simulink model "Analog_Digital_PID"  (R2025b)
settings: Solver=FixedStepAuto  StartTime=0.0  StopTime=inf  RelTol=1e-3  EnableMultiTasking=on
libraries: arduinolib x1, arduinoavrlib x1
settings Model: ExtModeTrigDuration=2  Creator=MSI  LastModifiedBy=MSI
settings SolverCC: AutoInsertRateTranBlk=on
settings OptimizationCC: EnhancedBackFolding=on  PassReuseOutputArgsAs=Individual arguments  ZeroExternalMemoryAtStartup=off  ZeroInternalMemoryAtStartup=off  MaxStackSize=64  OptimizeBlockOrder=speed  DifferentSizesBufferReuse=on  OptimizationCustomize=off  EfficientTunableParamExpr=on
settings DebuggingCC: ParameterTunabilityLossMsg=error
settings HardwareCC: ProdBitPerInt=16.0  ProdBitPerPointer=16.0  ProdBitPerSizeT=16.0  ProdBitPerPtrDiffT=16.0  ProdLargestAtomicFloat=None  ProdWordSize=8.0  ProdHWDeviceType=Atmel->AVR
settings SFSimCC: MATLABDynamicMemAlloc=off
settings RTWCC: SystemTargetFile=ert.tlc  HardwareBoard=Arduino Uno  TemplateMakefile=ert_default_tmf  Toolchain=Arduino AVR  BuildConfiguration=Faster Runs  Description=Embedded Coder
settings CodeAppCC: ForceParamTrailComments=on  IgnoreCustomStorageClasses=off  OperatorAnnotations=on  SimulinkDataObjDesc=on  SFDataObjDesc=on  InsertBlockDesc=on
settings ERTTargetCC: ExtModeTransport=3.0  ExtModeStaticAlloc=on  ExtModeAutomaticAllocSize=off  ExtModeStaticAllocSize=250.0  ExtModeMexFile=ext_xcp  ExtModeIntrfLevel=Level2 - Open  InlinedParameterPlacement=Hierarchical  SupportContinuousTime=on  SupportVariableSizeSignals=on

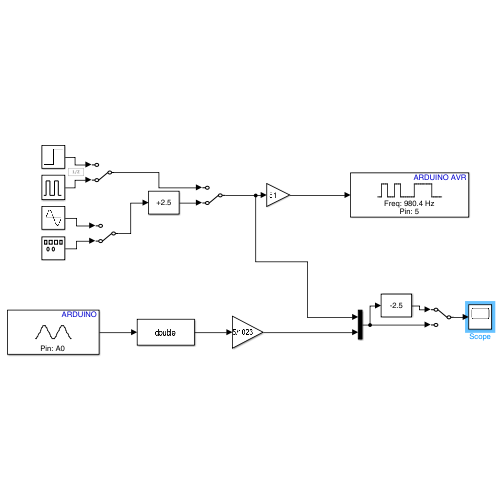
[thumbnail: Simulink's stored preview of the top-level diagram]
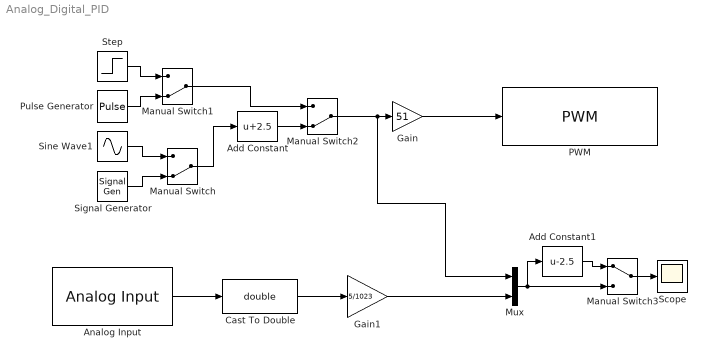
== system Analog_Digital_PID ==
  Add Constant : Bias  Bias=2.5  SaturateOnIntegerOverflow=off
  Add Constant1 : Bias  Bias=-2.5  SaturateOnIntegerOverflow=off
  Analog Input : arduinolib/Analog Input  pinNumber=0  ReadResultsOnly=off  ConversionTriggerSource=Software  ExternalTriggerType=uint32( 0 )  OutputDataType=uint16  EnableConversionCompleteNotify=off  EnableOuputStatus=off  SampleTime=0.01  blockPlatform=arduino
  Cast To Double : DataTypeConversion  OutDataTypeStr=double  SaturateOnIntegerOverflow=off  RndMeth=Floor
  Gain : Gain  Gain=51
  Gain1 : Gain  Gain=5/1023
  Manual Switch : ManualSwitch  CurrentSetting=0
  Manual Switch1 : ManualSwitch  CurrentSetting=0
  Manual Switch2 : ManualSwitch  CurrentSetting=0
  Manual Switch3 : ManualSwitch
  Mux : Mux  Inputs=2
  PWM : arduinoavrlib/PWM  pinNumber=5  desiredFrequency=980.4  achievableFrequency=980.4  EnableCompareMatchInterrupt=off  EnableOverflowInterrupt=off
  Pulse Generator : DiscretePulseGenerator  PulseType=Time based  Amplitude=5  Period=4  PulseWidth=50
  Scope : Scope
      settings: ActiveDisplayYMinimum=0.54594465242270174  ActiveDisplayYMaximum=1.5449366782755996  DataLoggingVariableName=Bode_Pulse
  Signal Generator : SignalGenerator  WaveForm=square  Amplitude=1.5  Frequency=5  Units=rad/sec
  Sine Wave1 : Sin  Amplitude=2.5  Frequency=5  SampleTime=0
  Step : Step  After=5  SampleTime=0.01
  wires:
  Analog Input/1 -> Cast To Double/1
  Cast To Double/1 -> Gain1/1
  Gain1/1 -> Mux/2
  Gain/1 -> PWM/1
  Manual Switch2/1 -> Mux/1, Gain/1
  Signal Generator/1 -> Manual Switch/2
  Sine Wave1/1 -> Manual Switch/1
  Step/1 -> Manual Switch1/1
  Pulse Generator/1 -> Manual Switch1/2
  Manual Switch1/1 -> Manual Switch2/1
  Manual Switch3/1 -> Scope/1
  Add Constant1/1 -> Manual Switch3/1
  Mux/1 -> Manual Switch3/2, Add Constant1/1
  Manual Switch/1 -> Add Constant/1
  Add Constant/1 -> Manual Switch2/2
